simulink model "acoustic_input"  (R2015b)
settings: Solver=FixedStepAuto  StartTime=0.0  StopTime=inf  FixedStep=0.1  RelTol=1e-3
libraries: robotlib x1, realtime_pacer_lib x1
settings Model: Creator=saucer  LastModifiedBy=saucer

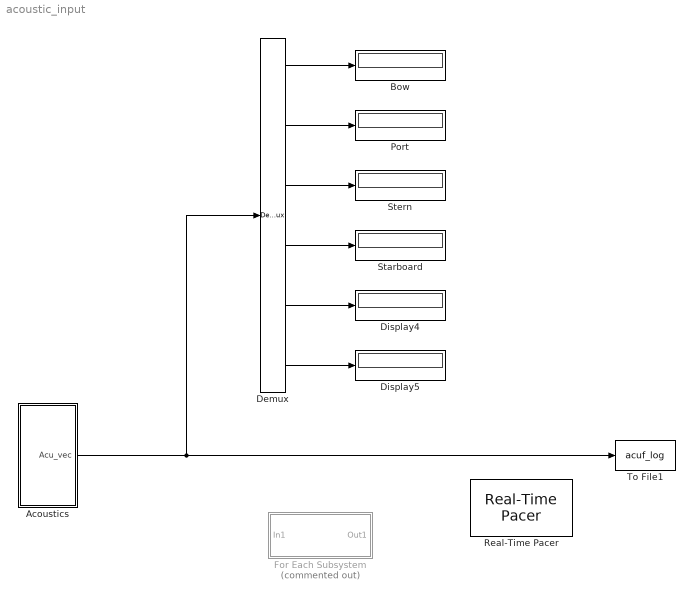
== system acoustic_input ==
  Acoustics : Subsystem
  Bow : Display
  Demux : Demux  Outputs=6
  Display4 : Display
  Display5 : Display
  For Each Subsystem : Subsystem  Commented=on  TreatAsAtomicUnit=on
  Port : Display
  Real-Time Pacer : realtime_pacer_lib/Real-Time Pacer  simTimePerRealTime=1
  Starboard : Display
  Stern : Display
  To File1 : ToFile  Filename=acuf_log  SaveFormat=Timeseries
  wires:
  Acoustics/1(Acu_vec) -> To File1/1, Demux/1
  Demux/1 -> Bow/1
  Demux/6 -> Display5/1
  Demux/5 -> Display4/1
  Demux/2 -> Port/1
  Demux/3 -> Stern/1
  Demux/4 -> Starboard/1

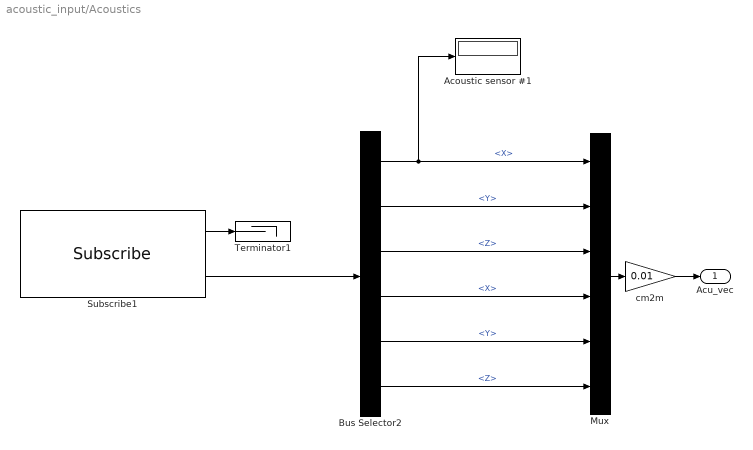
== system acoustic_input/Acoustics ==
  Acoustic sensor #1 : Display
  Bus Selector2 : BusSelector  OutputSignals=Linear.X,Linear.Y,Linear.Z,Angular.X,Angular.Y,Angular.Z
  Mux : Mux  Inputs=6
  Subscribe1 : robotlib/Subscribe  SourceLibraryInfo=This block requires Robotics System Toolbox  topicSource=Select from ROS network  topic=/Acoustics  messageType=geometry_msgs/Twist  sampleTime=-1  messageQueueLength=1
  Terminator1 : Terminator
  cm2m : Gain  Gain=0.01
  Acu_vec : Outport
  wires:
  Subscribe1/1 -> Terminator1/1
  Subscribe1/2 -> Bus Selector2/1
  Bus Selector2/1 -> Mux/1, Acoustic sensor #1/1  "<X>"
  Bus Selector2/6 -> Mux/6  "<Z>"
  Bus Selector2/5 -> Mux/5  "<Y>"
  Bus Selector2/4 -> Mux/4  "<X>"
  Bus Selector2/3 -> Mux/3  "<Z>"
  Bus Selector2/2 -> Mux/2  "<Y>"
  Mux/1 -> cm2m/1
  cm2m/1 -> Acu_vec/1

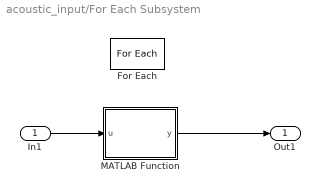
== system acoustic_input/For Each Subsystem ==
  In1 : Inport  Partition=on  PartitionDimension=1  PartitionWidth=1
  For Each : ForEach  DisableCoverage=on  IndexMode=One-based
  MATLAB Function : MATLAB Function  TreatAsAtomicUnit=on
  Out1 : Outport  ConcatenationDimension=1
  wires:
  In1/1 -> MATLAB Function/1(u)
  MATLAB Function/1(y) -> Out1/1

== matlab function acoustic_input/For Each Subsystem/MATLAB Function ==
  data: u input; y output
function y = fcn(u)
persistent u_old
if isempty(u_old)
    u_old = 0;
    y = u;
elseif abs(u-u_old) > 0.5
    y = u_old;
else
    u_old = u;
    y = u;
end
